simulink model "AER821_Lab1_Part2"  (R2015b)
settings: Solver=ode1  StartTime=0.0  StopTime=int  FixedStep=0.001  RelTol=1e-3
values from neighbouring files (symbols this model uses):
  Beq = 0    [Set_SRV02_Configuration.m]
  Eff_G = 0.9    [Set_SRV02_Configuration.m]
  Eff_M = 0.69    [Set_SRV02_Configuration.m]
  Jeq = Jeq + Jload    (= 0)    [Set_SRV02_Configuration.m]
  K_CABLE = 1    [Setup_SRV02_Aero_position.m]
  K_ENC = 0    [Set_SRV02_Configuration.m]
  Kg = 0    [Set_SRV02_Configuration.m]
  Km = 0.804e-3 * K_RDPS2RPM    [Set_SRV02_Configuration.m]
  Kt = 1.088 * K_OZ2N * K_IN2M    [Set_SRV02_Configuration.m]
  Rm = 2.6    [Set_SRV02_Configuration.m]
  VMAX_UPM = 0    [Set_SRV02_Configuration.m]
undefined symbols (not defined in the file or in its folder): HIL, qc_get_step_size
libraries: simulink_extras x3, quarc_library x3
settings Model: SimulationMode=external  ExtModeTrigDuration=10000  Creator=Admin  LastModifiedBy=Admin
settings SolverCC: PositivePriorityOrder=on
settings DataIOCC: SaveFormat=Array  SignalLoggingSaveFormat=ModelDataLogs
settings OptimizationCC: ExpressionDepthLimit=2147483647
settings DebuggingCC: UnderspecifiedInitializationDetection=Classic  MergeDetectMultiDrivingBlocksExec=none  SolverPrmCheckMsg=warning  FcnCallInpInsideContextMsg=UseLocalSettings  StateNameClashWarn=warning
settings HardwareCC: ProdBitPerPointer=32  ProdLargestAtomicFloat=None  ProdIntDivRoundTo=Undefined  ProdEndianess=Unspecified  ProdWordSize=32  ProdHWDeviceType=32-bit Generic
settings RTWCC: SystemTargetFile=quarc_win64.tlc  TemplateMakefile=quarc_default_tmf  Description=QUARC Win64 Target
settings STFCustomTargetCC: GeneratePreprocessorConditionals=Use local settings  CPPClassGenCompliant=off
settings GRTTargetCC: ParMdlRefBuildCompliant=off  CompOptLevelCompliant=off  CombineOutputUpdateFcns=off  MatFileLogging=off  CPPClassGenCompliant=off  GRTInterface=on  UseToolchainInfoCompliant=off  ExtMode=on  ExtModeMexFile=quarc_comm
settings ConfigComp: CovModelRefEnable=Off

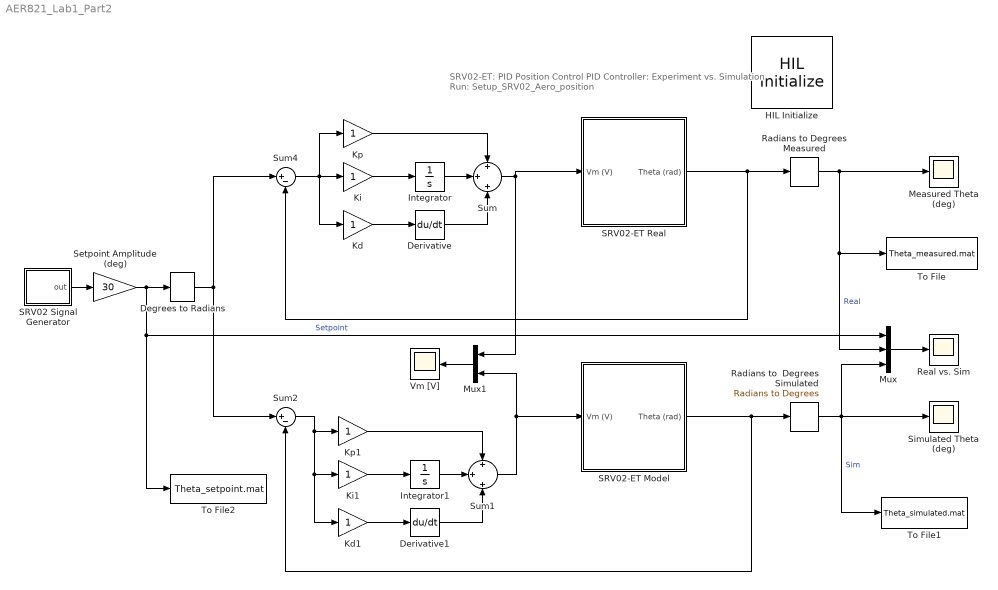
== system AER821_Lab1_Part2 ==
  note: SRV02-ET: PID Position Control
      | PID Controller: Experiment vs. Simulation
      | Run: Setup_SRV02_Aero_position
  Degrees to Radians : simulink_extras/Transformations/Degrees to Radians
  Derivative : Derivative
  Derivative1 : Derivative
  HIL Initialize : quarc_library/Data Acquisition/Generic/Configuration/HIL Initialize  object_name=HIL-1  board_type=q4  board_number=0  board_options=""  exclusive=off  active=off  hardware_clocks=[0:1]  clock_modes=[0 0]  initial_clock_frequencies=[]  set_clock_params_at_start=on  set_clock_params_at_switch_in=off  set_clock_frequencies_at_start=off  set_clock_frequencies_at_switch_in=off  analog_input_channels=[0:3]  analog_input_maximums=10  analog_input_minimums=-10  set_analog_input_params_at_start=off  set_analog_input_params_at_switch_in=off  analog_output_channels=[0:3]  analog_output_maximums=[10]  analog_output_minimums=[-10]  initial_analog_outputs=[0]  final_analog_outputs=[0]  watchdog_analog_outputs=0  set_analog_output_params_at_start=on  set_analog_output_params_at_switch_in=off  set_analog_outputs_at_start=on  set_analog_outputs_at_switch_in=off  set_analog_outputs_at_terminate=on  set_analog_outputs_at_switch_out=off  set_analog_outputs_on_watchdog=off  digital_input_channels=[]  digital_output_channels=[]  digital_output_configuration=[]  initial_digital_outputs=[1]  final_digital_outputs=[1]  watchdog_digital_outputs=[2]  set_digital_output_params_at_start=off  set_digital_output_params_at_switch_in=off  set_digital_outputs_at_start=on  set_digital_outputs_at_switch_in=off  set_digital_outputs_at_terminate=on  set_digital_outputs_at_switch_out=off  set_digital_outputs_on_watchdog=off  encoder_channels=[0:3]  quadrature=[4]  encoder_filter_frequency=(1/60e-9)/1  initial_encoder_counts=[0]  set_encoder_params_at_start=on  set_encoder_params_at_switch_in=off  set_encoder_counts_at_start=on  set_encoder_counts_at_switch_in=off  pwm_channels=[]  pwm_modes=[0]  pwm_frequency=(1/60e-9)/1024  pwm_configuration=[]  pwm_alignment=[]  pwm_polarity=[]  pwm_leading_deadband=[]  pwm_trailing_deadband=[]  initial_pwm_outputs=[0]  final_pwm_outputs=[0]  watchdog_pwm_outputs=[]  set_pwm_params_at_start=on  set_pwm_params_at_switch_in=off  set_pwm_outputs_at_start=on  set_pwm_outputs_at_switch_in=off  set_pwm_outputs_at_terminate=on  set_pwm_outputs_at_switch_out=off  set_pwm_outputs_on_watchdog=off  other_output_channels=[]  initial_other_outputs=[]  final_other_outputs=[]  watchdog_other_outputs=[]  set_other_outputs_at_start=off  set_other_outputs_at_switch_in=off  set_other_outputs_at_terminate=off  set_other_outputs_at_switch_out=off  set_other_outputs_on_watchdog=off
  Integrator : Integrator
  Integrator1 : Integrator
  Kd : Gain
  Kd1 : Gain
  Ki : Gain
  Ki1 : Gain
  Kp : Gain
  Kp1 : Gain
  Measured Theta (deg) : Scope
  Mux : Mux  Inputs=3
  Mux1 : Mux  Inputs=2
  Radians to  Degrees Simulated : simulink_extras/Transformations/Radians to Degrees
  Radians to Degrees Measured : simulink_extras/Transformations/Radians to Degrees
  "Real vs. Sim " : Scope
  SRV02 Signal Generator : Subsystem  mask(QET Signal Generator){sig_type=square, a=1, f=.4}
      mask prompts: sig_type "Signal Type"; a "Amplitude"; f "Frequency (Hz)"
      mask help: Generates a square, triangular, or sinusoidal waveform of a specified amplitude and frequency.
      mask Help: Choose the type of signal to be generated from the drop-down "Signal Type" box. Enter the amplitude and the frequency desired for the signal. Note: frequency is in Hertz.
      mask TypeOptions sig_type: square | triangle | sine
      mask Display: plot([0 1 1 2 2 3 4 5 6], [-1 -1 1 1 -1 -1 1 -1 -1])
  "SRV02-ET Model " : Subsystem
  "SRV02-ET Real " : Subsystem
  Setpoint Amplitude (deg) : Gain  Gain=30  SaturateOnIntegerOverflow=on  OutDataTypeStr=Inherit: Same as input  ParamDataTypeStr=Inherit: Same as input
  Simulated Theta (deg) : Scope
  Sum : Sum  Inputs=+|+|+
  Sum1 : Sum  Inputs=+|+|+
  Sum2 : Sum  Inputs=|+-  SaturateOnIntegerOverflow=on  InputSameDT=on  OutDataTypeStr=Inherit: Same as first input
  Sum4 : Sum  Inputs=|+-  SaturateOnIntegerOverflow=on  InputSameDT=on  OutDataTypeStr=Inherit: Same as first input
  To File : ToFile  Filename=Theta_measured.mat  MatrixName=position_meas
  To File1 : ToFile  Filename=Theta_simulated.mat  MatrixName=position_sim
  To File2 : ToFile  Filename=Theta_setpoint.mat  MatrixName=setpoint
  Vm [V] : Scope
  wires:
  SRV02 Signal Generator/1(out) -> Setpoint Amplitude (deg)/1
  Setpoint Amplitude (deg)/1 -> Degrees to Radians/1, Mux/1, To File2/1  "Setpoint"
  Sum/1 -> "SRV02-ET Real "/1(Vm (V)), Mux1/1
  Sum1/1 -> Mux1/2, "SRV02-ET Model "/1(Vm (V))
  "SRV02-ET Model "/1(Theta (rad)) -> Radians to  Degrees Simulated/1, Sum2/2
  Degrees to Radians/1 -> Sum4/1, Sum2/1
  Radians to  Degrees Simulated/1 -> Simulated Theta (deg)/1, To File1/1, Mux/3  "Sim"
  "SRV02-ET Real "/1(Theta (rad)) -> Sum4/2, Radians to Degrees Measured/1
  Radians to Degrees Measured/1 -> Measured Theta (deg)/1, Mux/2, To File/1  "Real"
  Mux/1 -> "Real vs. Sim "/1
  Mux1/1 -> Vm [V]/1
  Sum4/1 -> Kd/1, Kp/1, Ki/1
  Ki/1 -> Integrator/1
  Kd/1 -> Derivative/1
  Integrator/1 -> Sum/2
  Kp/1 -> Sum/1
  Derivative/1 -> Sum/3
  Sum2/1 -> Kd1/1, Ki1/1, Kp1/1
  Ki1/1 -> Integrator1/1
  Kd1/1 -> Derivative1/1
  Integrator1/1 -> Sum1/2
  Kp1/1 -> Sum1/1
  Derivative1/1 -> Sum1/3

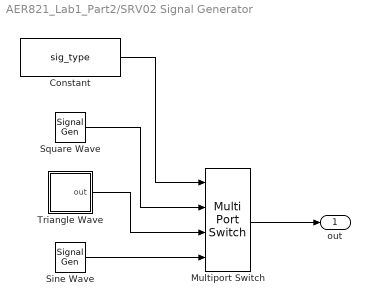
== system AER821_Lab1_Part2/SRV02 Signal Generator ==
  Constant : Constant  Value=sig_type
  Multiport Switch : MultiPortSwitch
  Sine Wave : SignalGenerator  Amplitude=a  Frequency=f
  Square Wave : SignalGenerator  WaveForm=square  Amplitude=a  Frequency=f
  Triangle Wave : Subsystem
  out : Outport
  wires:
  Constant/1 -> Multiport Switch/1
  Multiport Switch/1 -> out/1
  Sine Wave/1 -> Multiport Switch/4
  Triangle Wave/1(out) -> Multiport Switch/3
  Square Wave/1 -> Multiport Switch/2

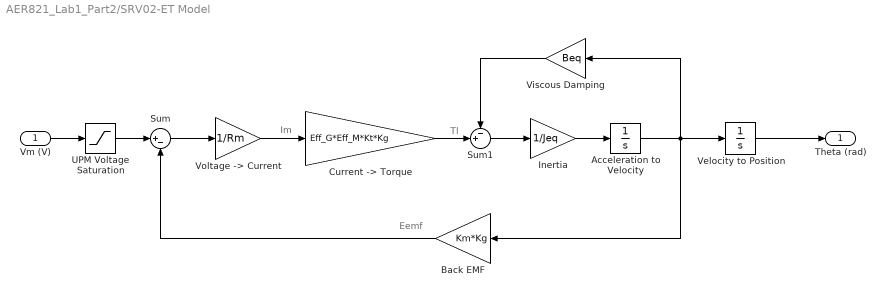
== system AER821_Lab1_Part2/SRV02-ET Model  ==
  note: Tl
  note: Im
  note: Eemf
  Vm (V) : Inport
  Acceleration to Velocity : Integrator
  Back EMF : Gain  Gain=Km*Kg  SaturateOnIntegerOverflow=on  OutDataTypeStr=Inherit: Same as input  ParamDataTypeStr=Inherit: Same as input
  "Current -> Torque" : Gain  Gain=Eff_G*Eff_M*Kt*Kg  SaturateOnIntegerOverflow=on  OutDataTypeStr=Inherit: Same as input  ParamDataTypeStr=Inherit: Same as input
  Inertia : Gain  Gain=1/Jeq  SaturateOnIntegerOverflow=on  OutDataTypeStr=Inherit: Same as input  ParamDataTypeStr=Inherit: Same as input
  Sum : Sum  Inputs=|+-  SaturateOnIntegerOverflow=on  InputSameDT=on  OutDataTypeStr=Inherit: Same as first input
  Sum1 : Sum  Inputs=-+|  SaturateOnIntegerOverflow=on  InputSameDT=on  OutDataTypeStr=Inherit: Same as first input
  "UPM Voltage Saturation " : Saturate  UpperLimit=VMAX_UPM  LowerLimit=-VMAX_UPM
  Velocity to Position : Integrator
  Viscous Damping : Gain  Gain=Beq  SaturateOnIntegerOverflow=on  OutDataTypeStr=Inherit: Same as input  ParamDataTypeStr=Inherit: Same as input
  "Voltage -> Current" : Gain  Gain=1/Rm  SaturateOnIntegerOverflow=on  OutDataTypeStr=Inherit: Same as input  ParamDataTypeStr=Inherit: Same as input
  Theta (rad) : Outport
  wires:
  Velocity to Position/1 -> Theta (rad)/1
  Sum/1 -> "Voltage -> Current"/1
  Inertia/1 -> Acceleration to Velocity/1
  Back EMF/1 -> Sum/2
  Sum1/1 -> Inertia/1
  "Current -> Torque"/1 -> Sum1/2
  Viscous Damping/1 -> Sum1/1
  Vm (V)/1 -> "UPM Voltage Saturation "/1
  "UPM Voltage Saturation "/1 -> Sum/1
  "Voltage -> Current"/1 -> "Current -> Torque"/1
  Acceleration to Velocity/1 -> Velocity to Position/1, Back EMF/1, Viscous Damping/1

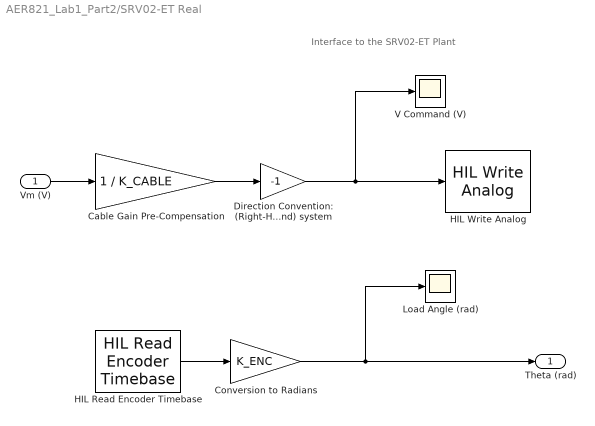
== system AER821_Lab1_Part2/SRV02-ET Real  ==
  note: Interface to the SRV02-ET Plant
  Vm (V) : Inport
  Cable Gain Pre-Compensation : Gain  Gain=1 / K_CABLE  SaturateOnIntegerOverflow=on  OutDataTypeStr=Inherit: Same as input  ParamDataTypeStr=Inherit: Same as input
  Conversion to Radians : Gain  Gain=K_ENC  SaturateOnIntegerOverflow=on  OutDataTypeStr=Inherit: Same as input  ParamDataTypeStr=Inherit: Same as input
  Direction Convention: (Right-Hand) system : Gain  Gain=-1  SaturateOnIntegerOverflow=on  OutDataTypeStr=Inherit: Same as input  ParamDataTypeStr=Inherit: Same as input
  HIL Read Encoder Timebase : quarc_library/Data Acquisition/Generic/Timebases/HIL Read Encoder Timebase  object_name=HIL-1  clock=0  channels=0  samples_in_buffer=max(ceil(1/qc_get_step_size), 1)  active=on  vector_output=off  data_type_mode=Inherit via back propagation  data_type=double
  HIL Write Analog : quarc_library/Data Acquisition/Generic/Immediate I//O/HIL Write Analog  object_name=HIL-1  channels=0  sample_time=-1  active=off  vector_input=off
  Load Angle (rad) : Scope
  V Command (V) : Scope
  Theta (rad) : Outport  InitialOutput=0
  wires:
  HIL Read Encoder Timebase/1 -> Conversion to Radians/1
  Vm (V)/1 -> Cable Gain Pre-Compensation/1
  Conversion to Radians/1 -> Theta (rad)/1, Load Angle (rad)/1
  Cable Gain Pre-Compensation/1 -> Direction Convention: (Right-Hand) system/1
  Direction Convention: (Right-Hand) system/1 -> HIL Write Analog/1, V Command (V)/1

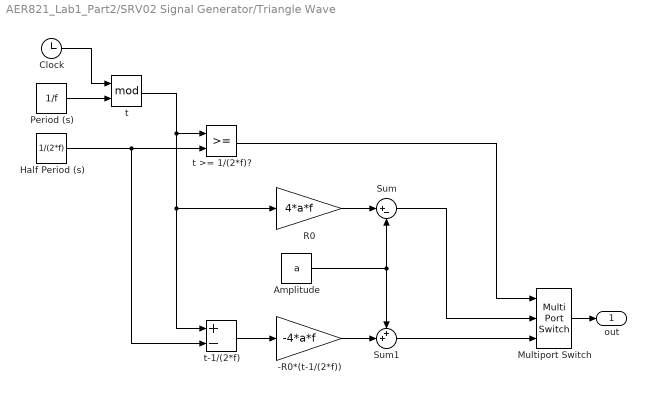
== system AER821_Lab1_Part2/SRV02 Signal Generator/Triangle Wave ==
  -R0*(t-1/(2*f)) : Gain  Gain=-4*a*f
  Amplitude : Constant  Value=a
  Clock : Clock
  Half Period (s) : Constant  Value=1/(2*f)
  Multiport Switch : MultiPortSwitch  DataPortOrder=Zero-based contiguous  Inputs=2  zeroidx=on
  Period (s) : Constant  Value=1/f
  R0 : Gain  Gain=4*a*f
  Sum : Sum  Inputs=|+-
  Sum1 : Sum  Inputs=++|
  t : Math  Operator=mod  SaturateOnIntegerOverflow=on
  t >= 1/(2*f)? : RelationalOperator  OutDataTypeStr=boolean
  t-1/(2*f) : Sum  Inputs=+-
  out : Outport
  wires:
  Multiport Switch/1 -> out/1
  Clock/1 -> t/1
  Period (s)/1 -> t/2
  t/1 -> t >= 1/(2*f)?/1, R0/1, t-1/(2*f)/1
  Half Period (s)/1 -> t >= 1/(2*f)?/2, t-1/(2*f)/2
  t-1/(2*f)/1 -> -R0*(t-1/(2*f))/1
  R0/1 -> Sum/1
  Amplitude/1 -> Sum/2, Sum1/1
  -R0*(t-1/(2*f))/1 -> Sum1/2
  t >= 1/(2*f)?/1 -> Multiport Switch/1
  Sum/1 -> Multiport Switch/2
  Sum1/1 -> Multiport Switch/3
